simulink model "SP_pitch_pid"  (Simulink 8.2)
settings: Solver=ode3  StartTime=0.0  StopTime=5  FixedStep=0.001  RelTol=1e-3
settings Model: Creator=Administrator  LastModifiedBy=zhaol
settings OptimizationCC: InitFltsAndDblsToZero=on

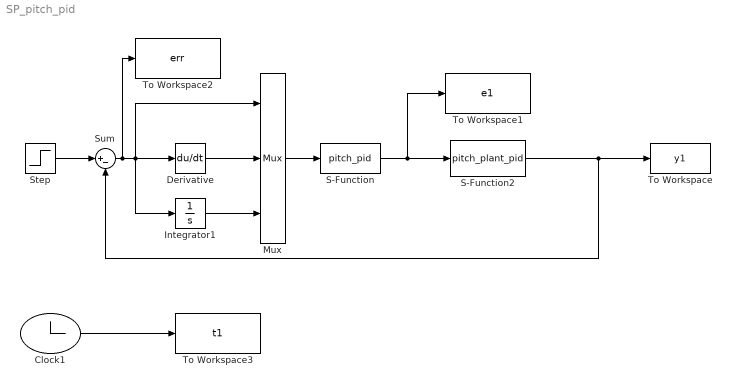
== system SP_pitch_pid ==
  Clock1 : Clock
  Derivative : Derivative
  Integrator1 : Integrator
  Mux : Mux  Inputs=3
  S-Function : S-Function  FunctionName=pitch_pid  EnableBusSupport=off
  S-Function2 : S-Function  FunctionName=pitch_plant_pid  EnableBusSupport=off
  Step : Step  After=0  SampleTime=0
  Sum : Sum  Inputs=|+-
  To Workspace : ToWorkspace  VariableName=y1  SampleTime=-1
  To Workspace1 : ToWorkspace  VariableName=e1  SampleTime=-1
  To Workspace2 : ToWorkspace  VariableName=err  SampleTime=-1
  To Workspace3 : ToWorkspace  VariableName=t1  SampleTime=-1
  wires:
  Clock1/1 -> To Workspace3/1
  Step/1 -> Sum/1
  Sum/1 -> To Workspace2/1, Mux/1, Integrator1/1, Derivative/1
  Derivative/1 -> Mux/2
  Integrator1/1 -> Mux/3
  Mux/1 -> S-Function/1
  S-Function/1 -> To Workspace1/1, S-Function2/1
  S-Function2/1 -> Sum/2, To Workspace/1
